simulink model "DCMotor_VelocityControl_Project"  (R2014a)
settings: Solver=ode45  StartTime=0.0  StopTime=0.015  RelTol=1e-3
settings Model: Creator=ABDULLAH  LastModifiedBy=Human Robotics

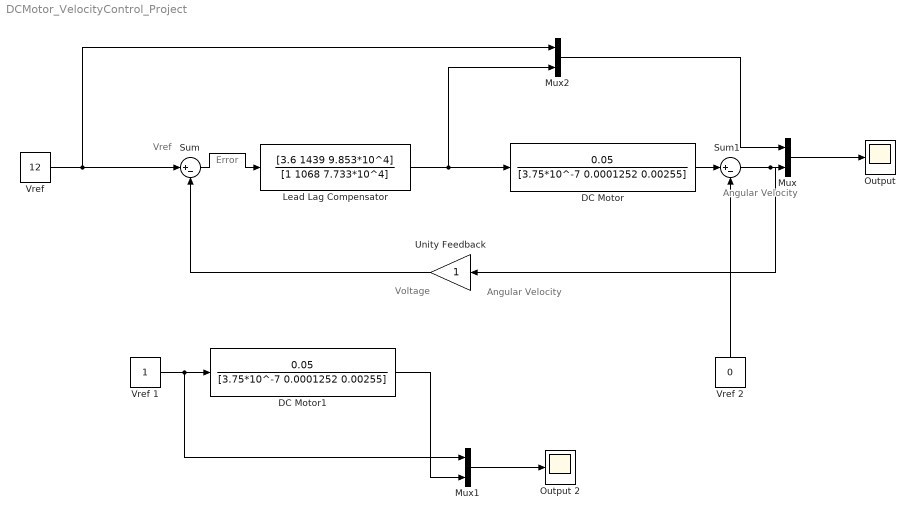
== system DCMotor_VelocityControl_Project ==
  note: Voltage
  note: Angular Velocity
  note: Angular
      | Velocity
  note: Error
  note: Vref
  DC Motor : TransferFcn  Numerator=[0.05]  Denominator=[3.75*10^-7 0.0001252 0.00255]
  DC Motor1 : TransferFcn  Numerator=[0.05]  Denominator=[3.75*10^-7 0.0001252 0.00255]
  "Lead Lag Compensator " : TransferFcn  Numerator=[3.6 1439 9.853*10^4]  Denominator=[1 1068 7.733*10^4]
  Mux : Mux  Inputs=2
  Mux1 : Mux  Inputs=2
  Mux2 : Mux  Inputs=2
  "Output " : Scope
  Output 2 : Scope
      settings: SaveName=ScopeData2
  Sum : Sum  Inputs=|+-
  Sum1 : Sum  Inputs=|+-
  Unity Feedback : Gain
  "Vref " : Constant  Value=12
  Vref 1 : Constant
  Vref 2 : Constant  Value=0
  wires:
  Mux/1 -> "Output "/1
  "Vref "/1 -> Mux2/1, Sum/1
  Unity Feedback/1 -> Sum/2
  Sum/1 -> "Lead Lag Compensator "/1
  Vref 1/1 -> Mux1/1, DC Motor1/1
  Mux1/1 -> Output 2/1
  DC Motor1/1 -> Mux1/2
  "Lead Lag Compensator "/1 -> Mux2/2, DC Motor/1
  DC Motor/1 -> Sum1/1
  Sum1/1 -> Unity Feedback/1, Mux/2
  Vref 2/1 -> Sum1/2
  Mux2/1 -> Mux/1
